simulink model "fin_pro_traj_sim"  (R2024b)
settings: Solver=ode4  StartTime=0.0  StopTime=20  FixedStep=0.005  RelTol=1e-3
values from neighbouring files (symbols this model uses):
  Bi = inv(hat_B)    [fin_pro_traj_mat.m]
  hat_A = [hat_a11 hat_a12; hat_a21 hat_a22]    [fin_pro_traj_mat.m]
  hat_B = [hat_b11 0; 0 hat_b22]    [fin_pro_traj_mat.m]
  hat_f1 = 0.900    (= 0.9)    [fin_pro_traj_mat.m]
  hat_f2 = 2.159    [fin_pro_traj_mat.m]
  k1 = 100    [fin_pro_traj_mat.m]
  k2 = 100    [fin_pro_traj_mat.m]
  Kd = 50    [fin_pro_traj_mat.m]
  Ki = 10    [fin_pro_traj_mat.m]
  Kp = 50    [fin_pro_traj_mat.m]
  lamda = 100    [fin_pro_traj_mat.m]
libraries: simulink x1
settings Model: Creator=wook9  LastModifiedBy=junso
settings RTWCC: GPUComputeCapability=3.5

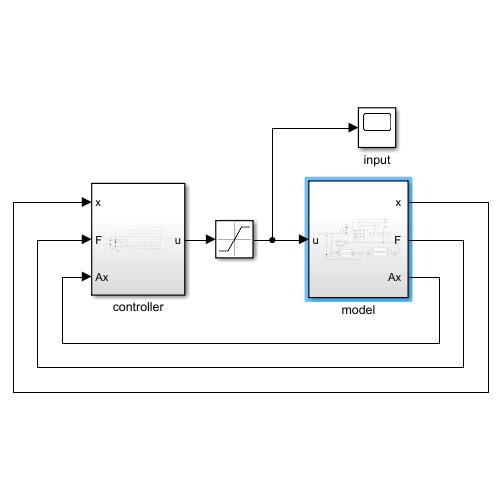
[thumbnail: Simulink's stored preview of the top-level diagram]
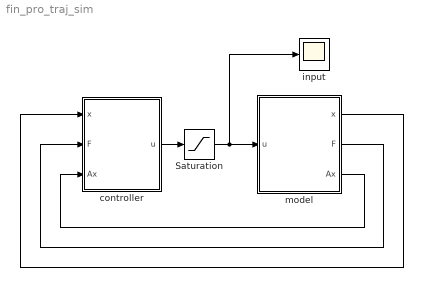
== system fin_pro_traj_sim ==
  Saturation : Saturate  UpperLimit=500  LowerLimit=-500
  controller : Subsystem
  input : Scope
  model : Subsystem
  wires:
  model/1("x ") -> controller/1(x)
  model/2("F ") -> controller/2(F)
  model/3("Ax ") -> controller/3(Ax)
  controller/1(u) -> Saturation/1
  Saturation/1 -> input/1, model/1(u)

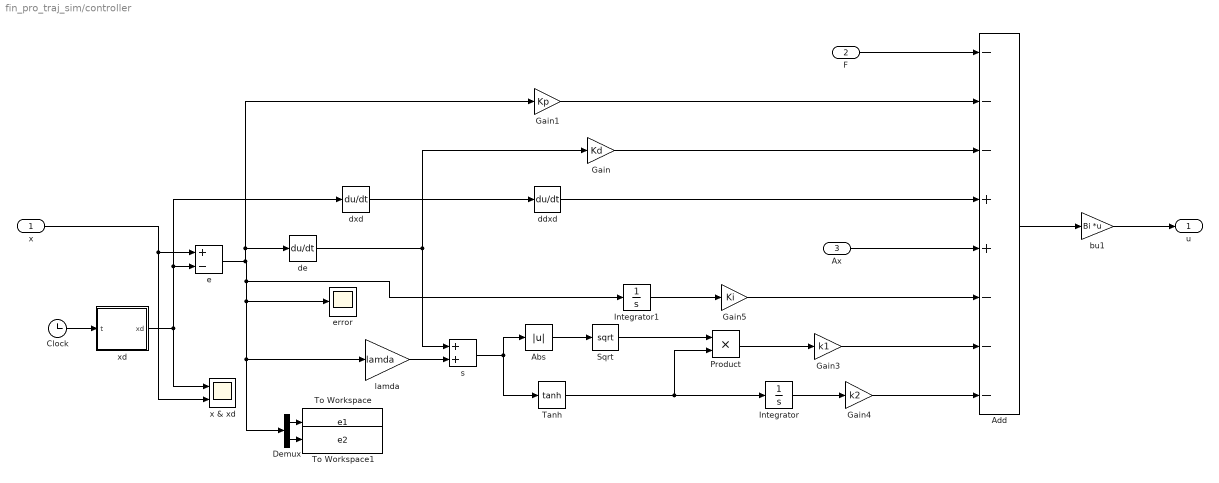
== system fin_pro_traj_sim/controller ==
  x : Inport
  F : Inport  Port=2
  Ax : Inport  Port=3
  Abs : Abs  SaturateOnIntegerOverflow=off
  Add : Sum  Inputs=---++---
  Clock : Clock
  Demux : Demux  Outputs=2
  Gain : Gain  Gain=Kd
  Gain1 : Gain  Gain=Kp
  Gain3 : Gain  Gain=k1
  Gain4 : Gain  Gain=k2
  Gain5 : Gain  Gain=Ki
  Integrator : Integrator
  Integrator1 : Integrator
  Product : Product
  Sqrt : Sqrt
  Tanh : Trigonometry  Operator=tanh
  To Workspace : ToWorkspace  VariableName=e1  SaveFormat=Timeseries  SampleTime=-1
  To Workspace1 : ToWorkspace  VariableName=e2  SaveFormat=Timeseries  SampleTime=-1
  bu1 : Gain  Gain=Bi  Multiplication=Matrix(K*u) (u vector)
  ddxd : Derivative
  de : Derivative
  dxd : Derivative
  e : Sum  Inputs=+-
  error : Scope
  lamda : Gain  Gain=lamda
  s : Sum
  x & xd : Scope  NumInputPorts=2
  xd : MATLAB Function  TreatAsAtomicUnit=on
  u : Outport
  wires:
  Clock/1 -> xd/1(t)
  e/1 -> Gain1/1, de/1, Integrator1/1, error/1, Demux/1, lamda/1
  xd/1(xd) -> dxd/1, e/2, x & xd/1
  Demux/1 -> To Workspace/1
  Demux/2 -> To Workspace1/1
  dxd/1 -> ddxd/1
  ddxd/1 -> Add/4
  lamda/1 -> s/2
  de/1 -> s/1, Gain/1
  F/1 -> Add/1
  x/1 -> x & xd/2, e/1
  Sqrt/1 -> Product/1
  Product/1 -> Gain3/1
  Gain3/1 -> Add/7
  Add/1 -> bu1/1
  Integrator/1 -> Gain4/1
  Gain4/1 -> Add/8
  Integrator1/1 -> Gain5/1
  Ax/1 -> Add/5
  Gain/1 -> Add/3
  Gain1/1 -> Add/2
  Gain5/1 -> Add/6
  s/1 -> Tanh/1, Abs/1
  Abs/1 -> Sqrt/1
  Tanh/1 -> Product/2, Integrator/1
  bu1/1 -> u/1

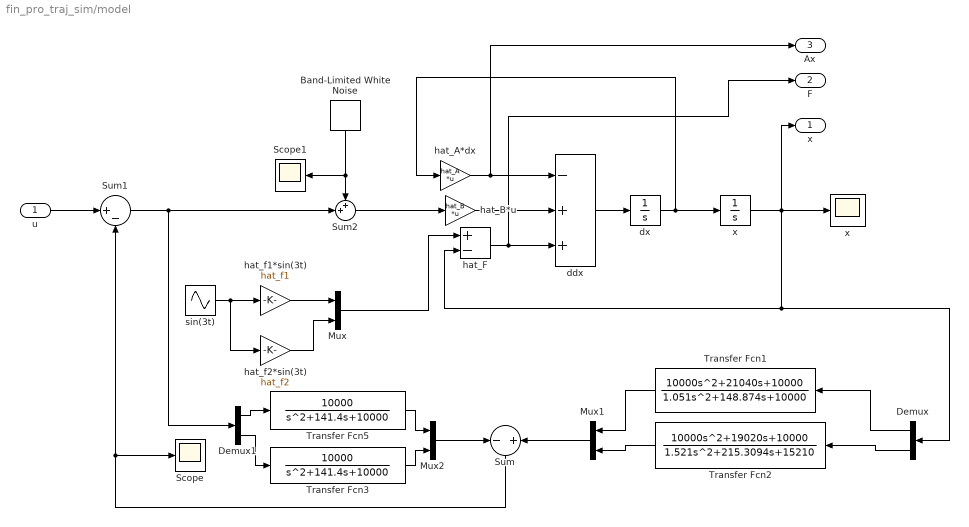
== system fin_pro_traj_sim/model ==
  u : Inport
  " x " : Scope
  Band-Limited White Noise : simulink/Sources/Band-Limited White Noise  Cov=[500]  Ts=0.005  seed=[23341]
  Demux : Demux  Outputs=2
  Demux1 : Demux  Outputs=2
  Mux : Mux  Inputs=2
  Mux1 : Mux  Inputs=2
  Mux2 : Mux  Inputs=2
  Scope : Scope
  Scope1 : Scope
  Sum : Sum  Inputs=-|+
  Sum1 : Sum  Inputs=|+-
  Sum2 : Sum  Inputs=++|
  Transfer Fcn1 : TransferFcn  Numerator=[10000 21040 10000]  Denominator=[1.051 148.874 10000]
  Transfer Fcn2 : TransferFcn  Numerator=[10000 19020 10000]  Denominator=[1.521 215.3094 15210]
  Transfer Fcn3 : TransferFcn  Numerator=[10000]  Denominator=[1 141.4 10000]
  Transfer Fcn5 : TransferFcn  Numerator=[10000]  Denominator=[1 141.4 10000]
  ddx : Sum  Inputs=-++
  dx : Integrator  InitialCondition=[0; 0]
  hat_A*dx : Gain  Gain=hat_A  Multiplication=Matrix(K*u) (u vector)
  hat_B*u : Gain  Gain=hat_B  Multiplication=Matrix(K*u) (u vector)
  hat_F : Sum  Inputs=+-
  hat_f1*sin(3t) : Gain  Gain=hat_f1
  hat_f2*sin(3t) : Gain  Gain=hat_f2
  sin(3t) : Sin  Frequency=3  SampleTime=0
  x : Integrator  InitialCondition=[0; 0]
  "x " : Outport
  "F " : Outport  Port=2
  "Ax " : Outport  Port=3
  wires:
  dx/1 -> x/1, hat_A*dx/1
  hat_A*dx/1 -> ddx/1, "Ax "/1
  ddx/1 -> dx/1
  Mux/1 -> hat_F/1
  hat_B*u/1 -> ddx/2
  hat_f2*sin(3t)/1 -> Mux/2
  hat_f1*sin(3t)/1 -> Mux/1
  sin(3t)/1 -> hat_f1*sin(3t)/1, hat_f2*sin(3t)/1
  x/1 -> "x "/1, " x "/1, Demux/1, hat_F/2
  hat_F/1 -> "F "/1, ddx/3
  u/1 -> Sum1/1
  Demux1/1 -> Transfer Fcn5/1
  Demux1/2 -> Transfer Fcn3/1
  Transfer Fcn5/1 -> Mux2/1
  Transfer Fcn3/1 -> Mux2/2
  Sum2/1 -> hat_B*u/1
  Mux2/1 -> Sum/1
  Sum1/1 -> Sum2/2, Demux1/1
  Mux1/1 -> Sum/2
  Transfer Fcn2/1 -> Mux1/2
  Transfer Fcn1/1 -> Mux1/1
  Sum/1 -> Scope/1, Sum1/2
  Demux/1 -> Transfer Fcn1/1
  Demux/2 -> Transfer Fcn2/1
  Band-Limited White Noise/1 -> Scope1/1, Sum2/1

== matlab function fin_pro_traj_sim/controller/xd ==
  data: t input; xd output
function xd = fcn(t)
    xd = [1*sin(20*t)+5*cos(3*t); -1*sin(20*t)-5*cos(3*t)];
end
